simulink model "distributed_swarm_controller"  (R2018a)
settings: Solver=VariableStepAuto  StartTime=0.0  StopTime=Inf  FixedStep=0.01  RelTol=1e-3  EnableMultiTasking=on
model workspace (MAT data in the model file):
  SL_ROS_VariableLengthArrays_MaxSizes.CommonInfo.ArrayTruncateAction = 'EmitWarning'
  SL_ROS_VariableLengthArrays_MaxSizes.MsgTypeMap = containers.Map
  SL_ROS_VariableLengthArrays_MaxSizes.MsgTypeMap.serialization.keys = {'sensor_msgs/Image', 'sensor_msgs/LaserScan'}
  SL_ROS_VariableLengthArrays_MaxSizes.MsgTypeMap.serialization.values{1}(1).PropertyName = 'Data'
  SL_ROS_VariableLengthArrays_MaxSizes.MsgTypeMap.serialization.values{1}(1).DataType = 'uint8'
  SL_ROS_VariableLengthArrays_MaxSizes.MsgTypeMap.serialization.values{1}(1).MaxLength = 691200
  SL_ROS_VariableLengthArrays_MaxSizes.MsgTypeMap.serialization.values{1}(2).PropertyName = 'Encoding'
  SL_ROS_VariableLengthArrays_MaxSizes.MsgTypeMap.serialization.values{1}(2).DataType = 'uint8'
  SL_ROS_VariableLengthArrays_MaxSizes.MsgTypeMap.serialization.values{1}(2).MaxLength = 128
  SL_ROS_VariableLengthArrays_MaxSizes.MsgTypeMap.serialization.values{2}(1).PropertyName = 'Intensities'
  SL_ROS_VariableLengthArrays_MaxSizes.MsgTypeMap.serialization.values{2}(1).DataType = 'single'
  SL_ROS_VariableLengthArrays_MaxSizes.MsgTypeMap.serialization.values{2}(1).MaxLength = 1081
  SL_ROS_VariableLengthArrays_MaxSizes.MsgTypeMap.serialization.values{2}(2).PropertyName = 'Ranges'
  SL_ROS_VariableLengthArrays_MaxSizes.MsgTypeMap.serialization.values{2}(2).DataType = 'single'
  SL_ROS_VariableLengthArrays_MaxSizes.MsgTypeMap.serialization.values{2}(2).MaxLength = 1081
  SL_ROS_VariableLengthArrays_MaxSizes.MsgTypeMap.serialization.uniformity = 0
  SL_ROS_VariableLengthArrays_MaxSizes.MsgTypeMap.serialization.keyType = 'char'
  SL_ROS_VariableLengthArrays_MaxSizes.MsgTypeMap.serialization.valueType = 'any'
undefined symbols (not defined in the file or in its folder): DiscIntNeverNeededParam, Vector_
libraries: robotlib x4, simulink x4, sharedTrackingLibrary x4, aerolibanimutils x1
settings Model: Creator=The MathWorks, Inc.  LastModifiedBy=Kevin_ME813
settings DataIOCC: LimitDataPoints=on  SaveFormat=Array
settings OptimizationCC: LifeSpan=Inf  MaxStackSize=64
settings DebuggingCC: SolverPrmCheckMsg=warning  SFUnexpectedBacktrackingDiag=warning  SFNoUnconditionalDefaultTransitionDiag=warning  SFExecutionAtInitializationDiag=none
settings HardwareCC: ProdBitPerPointer=32  ProdBitPerSizeT=32  ProdBitPerPtrDiffT=32  ProdLargestAtomicFloat=None  ProdIntDivRoundTo=Undefined  ProdEndianess=Unspecified  ProdWordSize=32  ProdHWDeviceType=Generic->Unspecified (assume 32-bit Generic)  UseEmbeddedCoderFeatures=off
settings ModelReferenceCC: PropagateSignalLabelsOutOfModel=off
settings RTWCC: SystemTargetFile=ert.tlc  HardwareBoard=Robot Operating System (ROS)  TLCOptions=-aInlineSetEventsForThisBaseRateFcn=TLC_FALSE -aSuppressMultiTaskScheduler=TLC_FALSE -aRateBasedStepFcn=0  TemplateMakefile=ert_default_tmf  Toolchain=Catkin  TargetLang=C++
settings CodeAppCC: StateflowObjectComments=on
settings ERTTargetCC: MultiwordLength=2048  ERTCustomFileBanners=off  SupportContinuousTime=on  SupportNonInlinedSFcns=on  RemoveResetFunc=off  SupportVariableSizeSignals=on  ModelStepFunctionPrototypeControlCompliant=off  ConvertIfToSwitch=off  SuppressUnreachableDefaultCases=off
settings ConfigComp: CovMetricSettings=dw  CovHtmlReporting=on  CovSaveCumulativeToWorkspaceVar=on  CovSaveSingleToWorkspaceVar=on  CovExternalEMLEnable=off  CovSFcnEnable=off

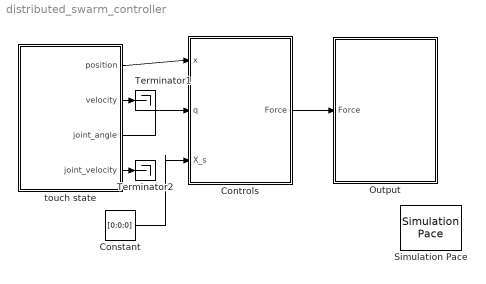
== system distributed_swarm_controller ==
  Constant : Constant  Value=[0;0;0]  SampleTime=0.01
  Controls : Subsystem
  Output : Subsystem
  Simulation Pace : aerolibanimutils/Simulation Pace  SimulationPace=1  SleepMode=MATLAB Thread  OutputPaceError=off  SampleTime=-1
  Terminator1 : Terminator
  Terminator2 : Terminator
  touch state : Subsystem
  wires:
  Controls/1(Force) -> Output/1(Force)
  touch state/1(position) -> Controls/1(x)
  touch state/3(joint_angle) -> Controls/2(q)
  Constant/1 -> Controls/3(X_s)
  touch state/2(velocity) -> Terminator1/1
  touch state/4(joint_velocity) -> Terminator2/1

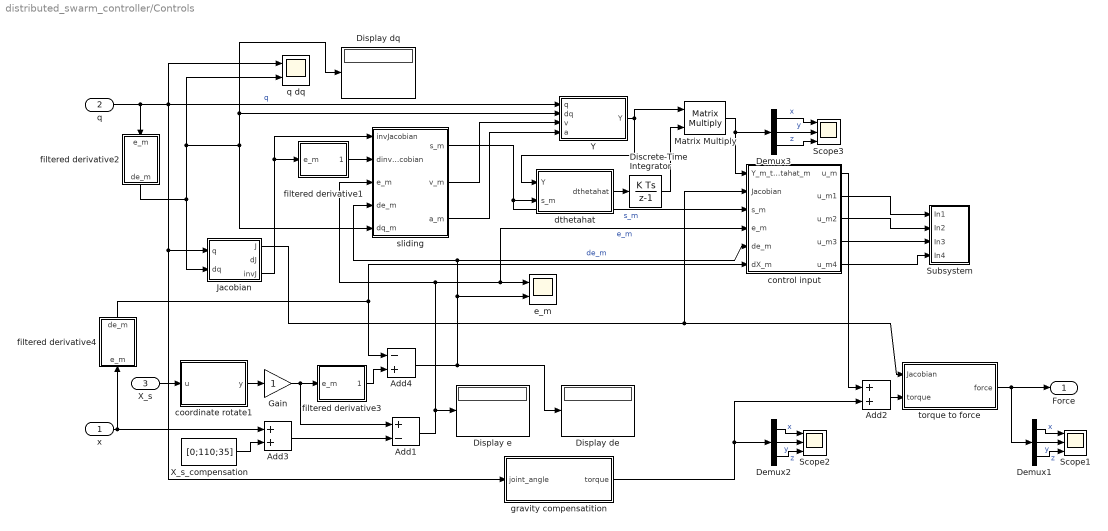
== system distributed_swarm_controller/Controls ==
  x : Inport
  q : Inport  Port=2
  X_s : Inport  Port=3
  Add1 : Sum  Inputs=+-
  Add2 : Sum
  Add3 : Sum
  Add4 : Sum  Inputs=-+
  Demux1 : Demux  Outputs=3
  Demux2 : Demux  Outputs=3
  Demux3 : Demux  Outputs=3
  Discrete-Time Integrator : DiscreteIntegrator  SampleTime=-1  ICPrevOutput=DiscIntNeverNeededParam  ICPrevScaledInput=DiscIntNeverNeededParam
  Display de : Display
  Display dq : Display
  Display e : Display
  Gain : Gain
  Jacobian : MATLAB Function  TreatAsAtomicUnit=on
  Matrix Multiply : Product  Multiplication=Matrix(*)
  Scope1 : Scope  NumInputPorts=3
  Scope2 : Scope  NumInputPorts=3
  Scope3 : Scope  NumInputPorts=3
  Subsystem : Subsystem
  X_s_compensation : Constant  Value=[0;110;35]  SampleTime=0.01
  Y : MATLAB Function  TreatAsAtomicUnit=on
  control input : MATLAB Function  TreatAsAtomicUnit=on
  coordinate rotate1 : MATLAB Function  TreatAsAtomicUnit=on
  dthetahat : MATLAB Function  TreatAsAtomicUnit=on
  e_m : Scope  NumInputPorts=2
  filtered derivative1 : Subsystem
  filtered derivative2 : Subsystem
  filtered derivative3 : Subsystem
  filtered derivative4 : Subsystem
  gravity compensatition : MATLAB Function  TreatAsAtomicUnit=on
  q dq : Scope  NumInputPorts=2
  sliding : MATLAB Function  TreatAsAtomicUnit=on
  torque to force : MATLAB Function  TreatAsAtomicUnit=on
  Force : Outport
  wires:
  Jacobian/1(J) -> torque to force/1(Jacobian), control input/2(Jacobian)
  gravity compensatition/1(torque) -> Demux2/1, Add2/2
  torque to force/1(force) -> Demux1/1, Force/1
  Demux1/1 -> Scope1/1  "x"
  Demux1/3 -> Scope1/3  "z"
  Demux1/2 -> Scope1/2  "y"
  Demux2/2 -> Scope2/2  "y"
  Demux2/3 -> Scope2/3  "z"
  Demux2/1 -> Scope2/1  "x"
  sliding/1(s_m) -> dthetahat/2(s_m), control input/3(s_m)  "s_m"
  q/1 -> Y/1(q), q dq/1, gravity compensatition/1(joint_angle), Jacobian/1(q), filtered derivative2/1(e_m)  "q"
  dthetahat/1(dthetahat) -> Discrete-Time Integrator/1
  Y/1(Y) -> Matrix Multiply/1, dthetahat/1(Y)
  Discrete-Time Integrator/1 -> Matrix Multiply/2
  filtered derivative2/1(de_m) -> Jacobian/2(dq), Display dq/1, Y/2(dq), sliding/5(dq_m), q dq/2
  X_s/1 -> coordinate rotate1/1(u)
  Gain/1 -> filtered derivative3/1(e_m), Add1/1
  coordinate rotate1/1(y) -> Gain/1
  x/1 -> Add3/1, filtered derivative4/1(e_m)
  Add1/1 -> Display e/1, control input/4(e_m), e_m/1, sliding/3(e_m)  "e_m"
  Add4/1 -> Display de/1, e_m/2, control input/5(de_m), sliding/4(de_m)  "de_m"
  control input/1(u_m) -> Add2/1
  Add2/1 -> torque to force/2(torque)
  X_s_compensation/1 -> Add3/2
  Add3/1 -> Add1/2
  filtered derivative3/1(de_m) -> Add4/2
  filtered derivative4/1(de_m) -> control input/6(dX_m), Add4/1
  sliding/2(v_m) -> Y/3(v)
  sliding/3(a_m) -> Y/4(a)
  Jacobian/3(invJ) -> filtered derivative1/1(e_m), sliding/1(invJacobian)
  filtered derivative1/1(de_m) -> sliding/2(dinvJacobian)
  Demux3/2 -> Scope3/2  "y"
  Demux3/3 -> Scope3/3  "z"
  Demux3/1 -> Scope3/1  "x"
  Matrix Multiply/1 -> control input/1(Y_m_thetahat_m), Demux3/1
  control input/2(u_m1) -> Subsystem/1(In1)
  control input/3(u_m2) -> Subsystem/2(In2)
  control input/4(u_m3) -> Subsystem/3(In3)
  control input/5(u_m4) -> Subsystem/4(In4)

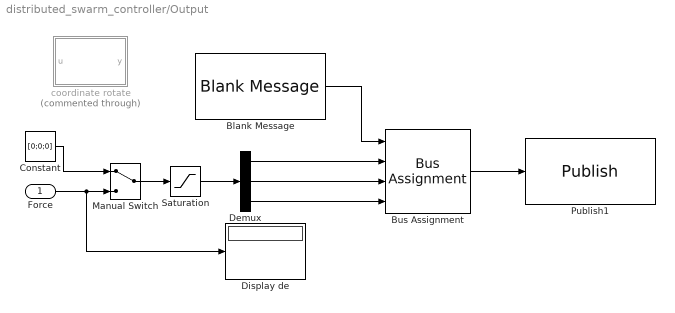
== system distributed_swarm_controller/Output ==
  Force : Inport
  Blank Message : robotlib/Blank Message  SourceLibraryInfo=This block requires Robotics System Toolbox  messageType=geometry_msgs/Vector3Stamped  SampleTime=0.01
      settings: SourceProductBaseCode=RO
  Bus Assignment : BusAssignment  DialogController=Simulink.DDGSource_BusAssignment  AssignedSignals=Vector_.X,Vector_.Y,Vector_.Z
  Constant : Constant  Value=[0;0;0]  SampleTime=0.01
  Demux : Demux  Outputs=3
  Display de : Display
  Manual Switch : ManualSwitch
  Publish1 : robotlib/Publish  SourceLibraryInfo=This block requires Robotics System Toolbox  topicSource=Select from ROS network  topic=/touch_1/touch_force  messageType=geometry_msgs/Vector3Stamped  messageQueueLength=105
      settings: SourceProductBaseCode=RO
  Saturation : Saturate  UpperLimit=[1;1;1]*5  LowerLimit=[-1;-1;-1]*5
  coordinate rotate : MATLAB Function  Commented=through  TreatAsAtomicUnit=on
  wires:
  Demux/2 -> Bus Assignment/3
  Demux/1 -> Bus Assignment/2
  Demux/3 -> Bus Assignment/4
  Bus Assignment/1 -> Publish1/1
  Blank Message/1 -> Bus Assignment/1
  Force/1 -> Display de/1, Manual Switch/2
  Constant/1 -> Manual Switch/1
  Manual Switch/1 -> Saturation/1
  Saturation/1 -> Demux/1

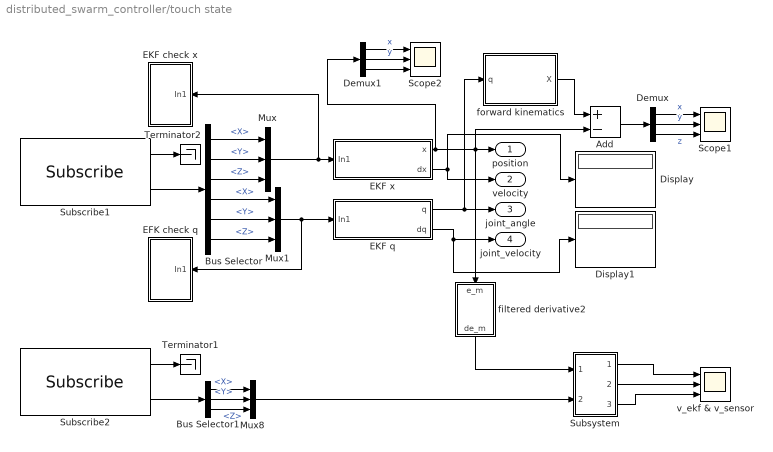
== system distributed_swarm_controller/touch state ==
  Add : Sum  Inputs=+-
  Bus Selector : BusSelector  DialogController=Simulink.DDGSource_BusSelector  OutputSignals=Twist.Linear.X,Twist.Linear.Y,Twist.Linear.Z,Twist.Angular.X,Twist.Angular.Y,Twist.Angular.Z
  Bus Selector1 : BusSelector  DialogController=Simulink.DDGSource_BusSelector  OutputSignals=Vector_.X,Vector_.Y,Vector_.Z
  Demux : Demux  Outputs=3
  Demux1 : Demux  Outputs=3
  Display : Display
  Display1 : Display
  EFK check q : Subsystem
  EKF check x : Subsystem
  EKF q : Subsystem
  EKF x : Subsystem
  Mux : Mux  Inputs=3
  Mux1 : Mux  Inputs=3
  Mux8 : Mux  Inputs=3
  Scope1 : Scope  NumInputPorts=3
  Scope2 : Scope  NumInputPorts=3
  Subscribe1 : robotlib/Subscribe  SourceLibraryInfo=This block requires Robotics System Toolbox  topicSource=Select from ROS network  topic=/touch_1/touch_state  messageType=geometry_msgs/TwistStamped  sampleTime=0.01  messageQueueLength=51
      settings: SourceProductBaseCode=RO
  Subscribe2 : robotlib/Subscribe  SourceLibraryInfo=This block requires Robotics System Toolbox  topicSource=Select from ROS network  topic=/touch_1/touch_vel_hd  messageType=geometry_msgs/Vector3Stamped  sampleTime=0.01  messageQueueLength=51
      settings: SourceProductBaseCode=RO
  Subsystem : Subsystem
  Terminator1 : Terminator
  Terminator2 : Terminator
  filtered derivative2 : Subsystem
  forward kinematics : MATLAB Function  TreatAsAtomicUnit=on
  v_ekf & v_sensor : Scope  NumInputPorts=3
  position : Outport
  velocity : Outport  Port=2
  joint_angle : Outport  Port=3
  joint_velocity : Outport  Port=4
  wires:
  Subscribe1/2 -> Bus Selector/1
  Bus Selector/1 -> Mux/1  "<X>"
  Bus Selector/5 -> Mux1/2  "<Y>"
  Bus Selector/4 -> Mux1/1  "<X>"
  Bus Selector/6 -> Mux1/3  "<Z>"
  Add/1 -> Demux/1
  Demux/3 -> Scope1/3  "z"
  Demux/1 -> Scope1/1  "x"
  Demux/2 -> Scope1/2  "y"
  Subscribe2/1 -> Terminator1/1
  Subscribe1/1 -> Terminator2/1
  Mux1/1 -> EFK check q/1(In1), EKF q/1(In1)
  Subscribe2/2 -> Bus Selector1/1
  forward kinematics/1(X) -> Add/1
  Bus Selector/2 -> Mux/2  "<Y>"
  Bus Selector/3 -> Mux/3  "<Z>"
  Mux/1 -> EKF x/1(In1), EKF check x/1(In1)
  EKF q/1(q) -> forward kinematics/1(q), joint_angle/1
  EKF x/2(dx) -> velocity/1, Display/1
  EKF q/2(dq) -> Display1/1, joint_velocity/1
  Subsystem/1(Out1) -> v_ekf & v_sensor/1
  Subsystem/2(Out2) -> v_ekf & v_sensor/2
  Subsystem/3(Out3) -> v_ekf & v_sensor/3
  Bus Selector1/1 -> Mux8/1  "<X>"
  Bus Selector1/2 -> Mux8/2  "<Y>"
  Bus Selector1/3 -> Mux8/3  "<Z>"
  Mux8/1 -> Subsystem/2(In2)
  filtered derivative2/1(de_m) -> Subsystem/1(In1)
  Demux1/2 -> Scope2/2  "y"
  Demux1/1 -> Scope2/1  "x"
  EKF x/1(x) -> Demux1/1, filtered derivative2/1(e_m), position/1, Add/2
  Demux1/3 -> Scope2/3

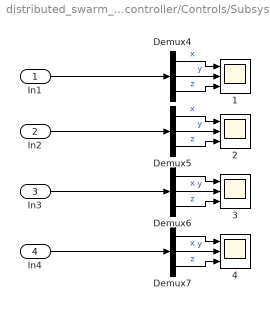
== system distributed_swarm_controller/Controls/Subsystem ==
  In1 : Inport
  In2 : Inport  Port=2
  In3 : Inport  Port=3
  In4 : Inport  Port=4
  {1..4} (4 alike) : Scope  NumInputPorts=3
  Demux{4..7} (4 alike) : Demux  Outputs=3
  wires:
  Demux5/1 -> 2/1  "x"
  Demux6/3 -> 3/3  "z"
  Demux6/1 -> 3/1  "x"
  In4/1 -> Demux7/1
  Demux5/3 -> 2/3  "z"
  Demux4/3 -> 1/3  "z"
  Demux6/2 -> 3/2  "y"
  Demux5/2 -> 2/2  "y"
  Demux4/2 -> 1/2  "y"
  Demux4/1 -> 1/1  "x"
  Demux7/1 -> 4/1  "x"
  Demux7/3 -> 4/3  "z"
  In2/1 -> Demux5/1
  Demux7/2 -> 4/2  "y"
  In3/1 -> Demux6/1
  In1/1 -> Demux4/1

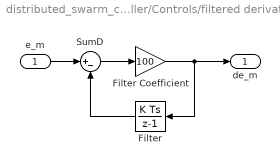
== system distributed_swarm_controller/Controls/filtered derivative1 ==
  e_m : Inport
  Filter : DiscreteIntegrator  DisableCoverage=on  SampleTime=-1  ICPrevOutput=DiscIntNeverNeededParam  ICPrevScaledInput=DiscIntNeverNeededParam
  Filter Coefficient : Gain  Gain=100
  SumD : Sum  DisableCoverage=on  Inputs=|+-
  de_m : Outport
  wires:
  e_m/1 -> SumD/1
  SumD/1 -> Filter Coefficient/1
  Filter/1 -> SumD/2
  Filter Coefficient/1 -> Filter/1, de_m/1

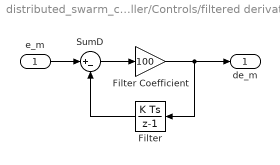
== system distributed_swarm_controller/Controls/filtered derivative2 ==
  e_m : Inport
  Filter : DiscreteIntegrator  DisableCoverage=on  SampleTime=-1  ICPrevOutput=DiscIntNeverNeededParam  ICPrevScaledInput=DiscIntNeverNeededParam
  Filter Coefficient : Gain  Gain=100
  SumD : Sum  DisableCoverage=on  Inputs=|+-
  de_m : Outport
  wires:
  Filter Coefficient/1 -> de_m/1, Filter/1
  Filter/1 -> SumD/2
  SumD/1 -> Filter Coefficient/1
  e_m/1 -> SumD/1

== system distributed_swarm_controller/Controls/filtered derivative3 ==
  e_m : Inport
  Filter : DiscreteIntegrator  DisableCoverage=on  SampleTime=-1  ICPrevOutput=DiscIntNeverNeededParam  ICPrevScaledInput=DiscIntNeverNeededParam
  Filter Coefficient : Gain  Gain=100
  SumD : Sum  DisableCoverage=on  Inputs=|+-
  de_m : Outport
  wires:
  Filter Coefficient/1 -> de_m/1, Filter/1
  Filter/1 -> SumD/2
  SumD/1 -> Filter Coefficient/1
  e_m/1 -> SumD/1

== system distributed_swarm_controller/Controls/filtered derivative4 ==
  e_m : Inport
  Filter : DiscreteIntegrator  DisableCoverage=on  SampleTime=-1  ICPrevOutput=DiscIntNeverNeededParam  ICPrevScaledInput=DiscIntNeverNeededParam
  Filter Coefficient : Gain  Gain=100
  SumD : Sum  DisableCoverage=on  Inputs=|+-
  de_m : Outport
  wires:
  e_m/1 -> SumD/1
  SumD/1 -> Filter Coefficient/1
  Filter/1 -> SumD/2
  Filter Coefficient/1 -> Filter/1, de_m/1

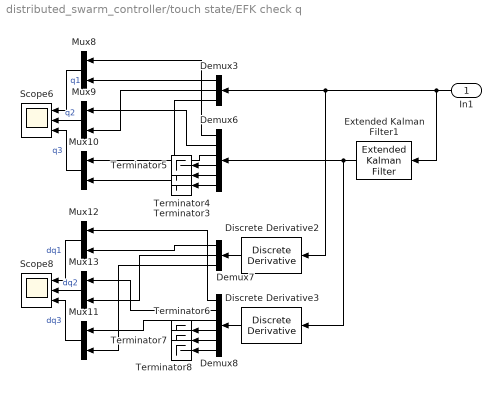
== system distributed_swarm_controller/touch state/EFK check q ==
  In1 : Inport
  Demux3 : Demux  Outputs=3
  Demux6 : Demux  Outputs=6
  Demux7 : Demux  Outputs=3
  Demux8 : Demux  Outputs=6
  Discrete Derivative2 : simulink/Discrete/Discrete Derivative  gainval=1.0  ICPrevScaledInput=0.0  OutMin=[]  OutMax=[]  OutDataType=fixdt(1, 16)  OutScaling=2^-10  DoSatur=off
  Discrete Derivative3 : simulink/Discrete/Discrete Derivative  gainval=1.0  ICPrevScaledInput=0.0  OutMin=[]  OutMax=[]  OutDataType=fixdt(1, 16)  OutScaling=2^-10  DoSatur=off
  Extended Kalman Filter1 : sharedTrackingLibrary/Extended Kalman Filter  StateTransitionFcn=myStateTransitionFcn  HasStateTransitionJacobianFcn=off  HasAdditiveProcessNoise=Additive  ProcessNoise=diag([0 0 0 1 1 1]*1e-3)  HasTimeVaryingProcessNoise=off  HasStateTransitionFcnExtraArgument=0  InitialState=[0 0 0 0 0 0]  InitialStateCovariance=1e-2  MeasurementFcn1=myMeasurementFcn  HasMeasurementJacobianFcn1=off  HasMeasurementEnablePort1=off  HasAdditiveMeasurementNoise1=Additive  MeasurementNoise1=diag([1;1;1]*1e-2)  HasTimeVaryingMeasurementNoise1=off  HasMeasurementFcnExtraArgument1=0  MeasurementFcn2=myMeasurementFcn  HasMeasurementJacobianFcn2=off  HasMeasurementEnablePort2=off  HasAdditiveMeasurementNoise2=Additive  MeasurementNoise2=1  HasTimeVaryingMeasurementNoise2=off  HasMeasurementFcnExtraArgument2=0  MeasurementFcn3=myMeasurementFcn  HasMeasurementJacobianFcn3=off  HasMeasurementEnablePort3=off  HasAdditiveMeasurementNoise3=Additive  MeasurementNoise3=1  HasTimeVaryingMeasurementNoise3=off  HasMeasurementFcnExtraArgument3=0  MeasurementFcn4=myMeasurementFcn  HasMeasurementJacobianFcn4=off  HasMeasurementEnablePort4=off  HasAdditiveMeasurementNoise4=Additive  MeasurementNoise4=1  HasTimeVaryingMeasurementNoise4=off  HasMeasurementFcnExtraArgument4=0  MeasurementFcn5=myMeasurementFcn  HasMeasurementJacobianFcn5=off  HasMeasurementEnablePort5=off  HasAdditiveMeasurementNoise5=Additive  MeasurementNoise5=1  HasTimeVaryingMeasurementNoise5=off  HasMeasurementFcnExtraArgument5=0  EnableMultirate=off  StateTransitionFcnSampleTime=1  MeasurementFcn1SampleTime=1  MeasurementFcn2SampleTime=1  MeasurementFcn3SampleTime=1  MeasurementFcn4SampleTime=1  MeasurementFcn5SampleTime=1  UseCurrentEstimator=on  OutputStateCovariance=off  DataType=double  SampleTime=0.01  NumberOfMeasurements=1
      settings: SourceProductName=Control System Toolbox  SourceProductBaseCode=CT
  Mux{8..13} (6 alike) : Mux  Inputs=2
  Scope6 : Scope  NumInputPorts=3
  Scope8 : Scope  NumInputPorts=3
  Terminator{3..8} (6 alike) : Terminator
  wires:
  In1/1 -> Discrete Derivative2/1, Demux3/1, Extended Kalman Filter1/1
  Demux3/1 -> Mux8/2
  Demux8/3 -> Mux11/1
  Demux3/2 -> Mux9/2
  Mux11/1 -> Scope8/3  "dq3"
  Mux12/1 -> Scope8/1  "dq1"
  Demux3/3 -> Mux10/2
  Demux7/2 -> Mux13/2
  Demux6/4 -> Terminator5/1
  Demux6/2 -> Mux9/1
  Demux8/5 -> Terminator7/1
  Demux8/4 -> Terminator6/1
  Mux13/1 -> Scope8/2  "dq2"
  Demux8/1 -> Mux12/1
  Mux9/1 -> Scope6/2  "q2"
  Mux10/1 -> Scope6/3  "q3"
  Demux6/3 -> Mux10/1
  Mux8/1 -> Scope6/1  "q1"
  Demux8/2 -> Mux13/1
  Demux6/1 -> Mux8/1
  Demux8/6 -> Terminator8/1
  Extended Kalman Filter1/1 -> Demux6/1, Discrete Derivative3/1
  Demux6/5 -> Terminator4/1
  Demux7/1 -> Mux12/2
  Demux7/3 -> Mux11/2
  Discrete Derivative2/1 -> Demux7/1
  Demux6/6 -> Terminator3/1
  Discrete Derivative3/1 -> Demux8/1

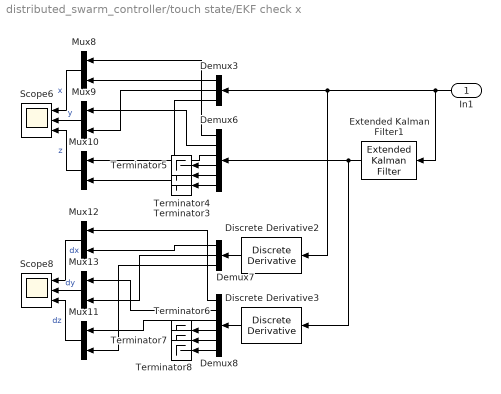
== system distributed_swarm_controller/touch state/EKF check x ==
  In1 : Inport
  Demux3 : Demux  Outputs=3
  Demux6 : Demux  Outputs=6
  Demux7 : Demux  Outputs=3
  Demux8 : Demux  Outputs=6
  Discrete Derivative2 : simulink/Discrete/Discrete Derivative  gainval=1.0  ICPrevScaledInput=0.0  OutMin=[]  OutMax=[]  OutDataType=fixdt(1, 16)  OutScaling=2^-10  DoSatur=off
  Discrete Derivative3 : simulink/Discrete/Discrete Derivative  gainval=1.0  ICPrevScaledInput=0.0  OutMin=[]  OutMax=[]  OutDataType=fixdt(1, 16)  OutScaling=2^-10  DoSatur=off
  Extended Kalman Filter1 : sharedTrackingLibrary/Extended Kalman Filter  StateTransitionFcn=myStateTransitionFcn  HasStateTransitionJacobianFcn=off  HasAdditiveProcessNoise=Additive  ProcessNoise=diag([0 0 0 1 1 1]*1e-3)  HasTimeVaryingProcessNoise=off  HasStateTransitionFcnExtraArgument=0  InitialState=[0 0 0 0 0 0]  InitialStateCovariance=1e-2  MeasurementFcn1=myMeasurementFcn  HasMeasurementJacobianFcn1=off  HasMeasurementEnablePort1=off  HasAdditiveMeasurementNoise1=Additive  MeasurementNoise1=diag([1;1;1]*1e-2)  HasTimeVaryingMeasurementNoise1=off  HasMeasurementFcnExtraArgument1=0  MeasurementFcn2=myMeasurementFcn  HasMeasurementJacobianFcn2=off  HasMeasurementEnablePort2=off  HasAdditiveMeasurementNoise2=Additive  MeasurementNoise2=1  HasTimeVaryingMeasurementNoise2=off  HasMeasurementFcnExtraArgument2=0  MeasurementFcn3=myMeasurementFcn  HasMeasurementJacobianFcn3=off  HasMeasurementEnablePort3=off  HasAdditiveMeasurementNoise3=Additive  MeasurementNoise3=1  HasTimeVaryingMeasurementNoise3=off  HasMeasurementFcnExtraArgument3=0  MeasurementFcn4=myMeasurementFcn  HasMeasurementJacobianFcn4=off  HasMeasurementEnablePort4=off  HasAdditiveMeasurementNoise4=Additive  MeasurementNoise4=1  HasTimeVaryingMeasurementNoise4=off  HasMeasurementFcnExtraArgument4=0  MeasurementFcn5=myMeasurementFcn  HasMeasurementJacobianFcn5=off  HasMeasurementEnablePort5=off  HasAdditiveMeasurementNoise5=Additive  MeasurementNoise5=1  HasTimeVaryingMeasurementNoise5=off  HasMeasurementFcnExtraArgument5=0  EnableMultirate=off  StateTransitionFcnSampleTime=1  MeasurementFcn1SampleTime=1  MeasurementFcn2SampleTime=1  MeasurementFcn3SampleTime=1  MeasurementFcn4SampleTime=1  MeasurementFcn5SampleTime=1  UseCurrentEstimator=on  OutputStateCovariance=off  DataType=double  SampleTime=0.01  NumberOfMeasurements=1
      settings: SourceProductName=Control System Toolbox  SourceProductBaseCode=CT
  Mux{8..13} (6 alike) : Mux  Inputs=2
  Scope6 : Scope  NumInputPorts=3
  Scope8 : Scope  NumInputPorts=3
  Terminator{3..8} (6 alike) : Terminator
  wires:
  Discrete Derivative3/1 -> Demux8/1
  Demux6/6 -> Terminator3/1
  Discrete Derivative2/1 -> Demux7/1
  Demux7/3 -> Mux11/2
  Demux7/1 -> Mux12/2
  Demux6/5 -> Terminator4/1
  Extended Kalman Filter1/1 -> Demux6/1, Discrete Derivative3/1
  Demux8/6 -> Terminator8/1
  Demux6/1 -> Mux8/1
  Demux8/2 -> Mux13/1
  Mux8/1 -> Scope6/1  "x"
  Demux6/3 -> Mux10/1
  Mux10/1 -> Scope6/3  "z"
  Mux9/1 -> Scope6/2  "y"
  Demux8/1 -> Mux12/1
  Mux13/1 -> Scope8/2  "dy"
  Demux8/4 -> Terminator6/1
  Demux8/5 -> Terminator7/1
  Demux6/2 -> Mux9/1
  Demux6/4 -> Terminator5/1
  Demux7/2 -> Mux13/2
  Demux3/3 -> Mux10/2
  Mux12/1 -> Scope8/1  "dx"
  Mux11/1 -> Scope8/3  "dz"
  Demux3/2 -> Mux9/2
  Demux8/3 -> Mux11/1
  Demux3/1 -> Mux8/2
  In1/1 -> Extended Kalman Filter1/1, Demux3/1, Discrete Derivative2/1

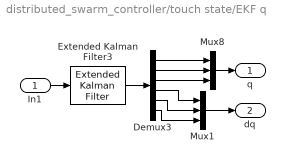
== system distributed_swarm_controller/touch state/EKF q ==
  In1 : Inport
  Demux3 : Demux  Outputs=6
  Extended Kalman Filter3 : sharedTrackingLibrary/Extended Kalman Filter  StateTransitionFcn=myStateTransitionFcn  HasStateTransitionJacobianFcn=off  HasAdditiveProcessNoise=Additive  ProcessNoise=diag([0 0 0 1 1 1]*5e-2)  HasTimeVaryingProcessNoise=off  HasStateTransitionFcnExtraArgument=0  InitialState=[0 0 0 0 0 0]  InitialStateCovariance=diag([1 1 1 1 1 1]*1e-1)  MeasurementFcn1=myMeasurementFcn  HasMeasurementJacobianFcn1=off  HasMeasurementEnablePort1=off  HasAdditiveMeasurementNoise1=Additive  MeasurementNoise1=diag([1;1;1]*3e-3)  HasTimeVaryingMeasurementNoise1=off  HasMeasurementFcnExtraArgument1=0  MeasurementFcn2=myMeasurementFcn  HasMeasurementJacobianFcn2=off  HasMeasurementEnablePort2=off  HasAdditiveMeasurementNoise2=Additive  MeasurementNoise2=1  HasTimeVaryingMeasurementNoise2=off  HasMeasurementFcnExtraArgument2=0  MeasurementFcn3=myMeasurementFcn  HasMeasurementJacobianFcn3=off  HasMeasurementEnablePort3=off  HasAdditiveMeasurementNoise3=Additive  MeasurementNoise3=1  HasTimeVaryingMeasurementNoise3=off  HasMeasurementFcnExtraArgument3=0  MeasurementFcn4=myMeasurementFcn  HasMeasurementJacobianFcn4=off  HasMeasurementEnablePort4=off  HasAdditiveMeasurementNoise4=Additive  MeasurementNoise4=1  HasTimeVaryingMeasurementNoise4=off  HasMeasurementFcnExtraArgument4=0  MeasurementFcn5=myMeasurementFcn  HasMeasurementJacobianFcn5=off  HasMeasurementEnablePort5=off  HasAdditiveMeasurementNoise5=Additive  MeasurementNoise5=1  HasTimeVaryingMeasurementNoise5=off  HasMeasurementFcnExtraArgument5=0  EnableMultirate=off  StateTransitionFcnSampleTime=1  MeasurementFcn1SampleTime=1  MeasurementFcn2SampleTime=1  MeasurementFcn3SampleTime=1  MeasurementFcn4SampleTime=1  MeasurementFcn5SampleTime=1  UseCurrentEstimator=on  OutputStateCovariance=off  DataType=double  SampleTime=0.01  NumberOfMeasurements=1
      settings: SourceProductName=Control System Toolbox  SourceProductBaseCode=CT
  Mux1 : Mux  Inputs=3
  Mux8 : Mux  Inputs=3
  q : Outport
  dq : Outport  Port=2
  wires:
  Mux8/1 -> q/1
  Demux3/6 -> Mux1/3
  Demux3/2 -> Mux8/2
  Demux3/3 -> Mux8/3
  Demux3/1 -> Mux8/1
  In1/1 -> Extended Kalman Filter3/1
  Demux3/4 -> Mux1/1
  Extended Kalman Filter3/1 -> Demux3/1
  Demux3/5 -> Mux1/2
  Mux1/1 -> dq/1

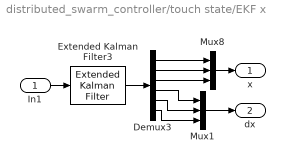
== system distributed_swarm_controller/touch state/EKF x ==
  In1 : Inport
  Demux3 : Demux  Outputs=6
  Extended Kalman Filter3 : sharedTrackingLibrary/Extended Kalman Filter  StateTransitionFcn=myStateTransitionFcn  HasStateTransitionJacobianFcn=off  HasAdditiveProcessNoise=Additive  ProcessNoise=diag([0 0 0 1 1 1]*5e-2)  HasTimeVaryingProcessNoise=off  HasStateTransitionFcnExtraArgument=0  InitialState=[4 -110 -35 0 0 0]  InitialStateCovariance=diag([2 1 2 1 1 1])  MeasurementFcn1=myMeasurementFcn  HasMeasurementJacobianFcn1=off  HasMeasurementEnablePort1=off  HasAdditiveMeasurementNoise1=Additive  MeasurementNoise1=diag([1;1;1]*3e-3)  HasTimeVaryingMeasurementNoise1=off  HasMeasurementFcnExtraArgument1=0  MeasurementFcn2=myMeasurementFcn  HasMeasurementJacobianFcn2=off  HasMeasurementEnablePort2=off  HasAdditiveMeasurementNoise2=Additive  MeasurementNoise2=1  HasTimeVaryingMeasurementNoise2=off  HasMeasurementFcnExtraArgument2=0  MeasurementFcn3=myMeasurementFcn  HasMeasurementJacobianFcn3=off  HasMeasurementEnablePort3=off  HasAdditiveMeasurementNoise3=Additive  MeasurementNoise3=1  HasTimeVaryingMeasurementNoise3=off  HasMeasurementFcnExtraArgument3=0  MeasurementFcn4=myMeasurementFcn  HasMeasurementJacobianFcn4=off  HasMeasurementEnablePort4=off  HasAdditiveMeasurementNoise4=Additive  MeasurementNoise4=1  HasTimeVaryingMeasurementNoise4=off  HasMeasurementFcnExtraArgument4=0  MeasurementFcn5=myMeasurementFcn  HasMeasurementJacobianFcn5=off  HasMeasurementEnablePort5=off  HasAdditiveMeasurementNoise5=Additive  MeasurementNoise5=1  HasTimeVaryingMeasurementNoise5=off  HasMeasurementFcnExtraArgument5=0  EnableMultirate=off  StateTransitionFcnSampleTime=1  MeasurementFcn1SampleTime=1  MeasurementFcn2SampleTime=1  MeasurementFcn3SampleTime=1  MeasurementFcn4SampleTime=1  MeasurementFcn5SampleTime=1  UseCurrentEstimator=on  OutputStateCovariance=off  DataType=double  SampleTime=0.01  NumberOfMeasurements=1
      settings: SourceProductName=Control System Toolbox  SourceProductBaseCode=CT
  Mux1 : Mux  Inputs=3
  Mux8 : Mux  Inputs=3
  x : Outport
  dx : Outport  Port=2
  wires:
  Demux3/5 -> Mux1/2
  Extended Kalman Filter3/1 -> Demux3/1
  Demux3/4 -> Mux1/1
  In1/1 -> Extended Kalman Filter3/1
  Demux3/1 -> Mux8/1
  Demux3/3 -> Mux8/3
  Demux3/2 -> Mux8/2
  Demux3/6 -> Mux1/3
  Mux8/1 -> x/1
  Mux1/1 -> dx/1

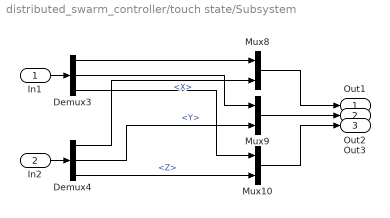
== system distributed_swarm_controller/touch state/Subsystem ==
  In1 : Inport
  In2 : Inport  Port=2
  Demux3 : Demux  Outputs=3
  Demux4 : Demux  Outputs=3
  Mux10 : Mux  Inputs=2
  Mux8 : Mux  Inputs=2
  Mux9 : Mux  Inputs=2
  Out1 : Outport
  Out2 : Outport  Port=2
  Out3 : Outport  Port=3
  wires:
  In2/1 -> Demux4/1
  Demux4/2 -> Mux9/2  "<Y>"
  Demux3/1 -> Mux8/1
  Demux4/1 -> Mux8/2  "<X>"
  Demux3/3 -> Mux10/1
  Demux3/2 -> Mux9/1
  Mux10/1 -> Out3/1
  Demux4/3 -> Mux10/2  "<Z>"
  Mux8/1 -> Out1/1
  Mux9/1 -> Out2/1
  In1/1 -> Demux3/1

== system distributed_swarm_controller/touch state/filtered derivative2 ==
  e_m : Inport
  Filter : DiscreteIntegrator  DisableCoverage=on  SampleTime=-1  ICPrevOutput=DiscIntNeverNeededParam  ICPrevScaledInput=DiscIntNeverNeededParam
  Filter Coefficient : Gain  Gain=100
  SumD : Sum  DisableCoverage=on  Inputs=|+-
  de_m : Outport
  wires:
  Filter Coefficient/1 -> de_m/1, Filter/1
  Filter/1 -> SumD/2
  SumD/1 -> Filter Coefficient/1
  e_m/1 -> SumD/1

== matlab function distributed_swarm_controller/Controls/torque to force ==
  data: Jacobian input; torque input; force output
function force = fcn(Jacobian, torque)

force = pinv(Jacobian).'*torque;

== matlab function distributed_swarm_controller/Controls/gravity compensatition ==
  data: joint_angle input; torque output
function torque = fcn(joint_angle)
q1 = joint_angle(1);
q2 = joint_angle(2);
q3 = joint_angle(3);
c1 = 85;
c2 = 70;

result = [0;c1*sin(q2+q3)+c2*cos(q2);c1*sin(q2+q3)];
% if result(2) < 0
%     result(2) = 0;
% end
torque = result;

== matlab function distributed_swarm_controller/touch state/forward kinematics ==
  data: q input; X output
function X = fcn(q)
%#codegen

l1=133;
l2=133;

q1 = q(1);
q2 = q(2);
q3 = q(3);

s1 = sin(q1);
s2 = sin(q2);
s3 = sin(q3);

c1 = cos(q1);
c2 = cos(q2);
c3 = cos(q3);

X1 = -l1*s1*c2 - l2*s1*s2*c3 - l2*s1*c2*s3;
X2 = l1*s2 - l2*c2*c3 + l2*s2*s3 + l2;
X3 = l1*c1*c2 - l1 + l2*c1*s2*c3 + l2*c1*c2*s3;

X = [ X1;
      X2;
      X3];

== matlab function distributed_swarm_controller/Output/coordinate rotate ==
  data: u input; y output
function y = fcn(u)

y = roty(-90)*rotx(-90)*u;

== matlab function distributed_swarm_controller/Controls/control input ==
  data: Y_m_thetahat_m input; Jacobian input; s_m input; e_m input; u_m output; de_m input; dX_m input; u_m1 output; u_m2 output; u_m3 output; u_m4 output
function [u_m, u_m1,u_m2, u_m3, u_m4] = fcn(Y_m_thetahat_m, Jacobian, s_m, e_m, de_m, dX_m)
k_sm = diag([15;20;20]);
k_pm = diag([1.7;2.5;2.5]*10^(-4));
k_dm = diag([1.7;1.5;1.5]*10^(-4));
k_tm = diag([1;1.5;1.5]*4);
p_m = -k_tm*e_m + dX_m;
% u_m = Y_m_thetahat_m ...
%     - (k_sm + k_pm*Jacobian.'*Jacobian)*s_m ...
%     + k_dm*Jacobian.'*de_m;
u_m1 = Y_m_thetahat_m;
u_m2 = - k_sm*s_m;
u_m3 = - k_pm*Jacobian.'*p_m;
u_m4 = k_dm*Jacobian.'*de_m;
u_m = u_m1 + u_m2 + u_m3 + u_m4;

== matlab function distributed_swarm_controller/Controls/sliding ==
  data: invJacobian input; dinvJacobian input; e_m input; de_m input; dq_m input; s_m output; v_m output; a_m output
function [s_m, v_m, a_m] = fcn(invJacobian, dinvJacobian, e_m, de_m, dq_m)
k_tm = diag([1;1.5;1.5]*4);
s_m = -invJacobian*k_tm*e_m + dq_m;
v_m = dq_m - s_m;
a_m = dinvJacobian*k_tm*e_m + invJacobian*k_tm*de_m;

== matlab function distributed_swarm_controller/Controls/Y ==
  data: q input; Y output; dq input; v input; a input
function Y = fcn(q,dq,v,a)
%#codegen

Y11=a(1)*cos(2*q(2))-sin(2*q(2))*(v(2)*dq(1)-v(1)*dq(2));
Y12=-sin(2*q(2)+2*q(3))*dq(1)*(v(2)+v(3))-v(1)*sin(2*q(2)+2*q(3))*(dq(2)-dq(3))+a(1)*cos(2*q(2)+2*q(3));
Y13=a(1)*(sin(2*q(2)+ q(3))+sin(q(3)))+0.5*cos(q(3))*(v(1)*dq(3)+v(3)*dq(1))+cos(2*q(2)+q(3))*(v(2)*dq(1)+0.5*v(3)*dq(1)+v(1)*dq(2)+0.5*v(1)*dq(3));
Y14=a(1);
Y15=0;
Y16=0;
Y17=0;
Y18=0;

Y21=v(1)*sin(2*q(2))*dq(1);
Y22=v(1)*sin(2*q(2)+2*q(3))*dq(1);
Y23=sin(q(3))*(2*a(2)+a(3))-v(1)*cos(2*q(2)+q(3))*dq(1)+cos(q(3))*(v(3)*dq(2)+v(3)*dq(3)+v(2)*dq(3));
Y24=0;
Y25=a(2);
Y26=a(3);
Y27=sin(q(2)+q(3));
Y28=cos(q(2));


Y31=0;
Y32=v(1)*sin(2*q(2)+2*q(3))*dq(1);
Y33=a(2)*sin(q(3))-(0.5*v(1)*cos(2*q(2)+q(3))+0.5*v(1)*cos(q(3)))*dq(1)-cos(q(3))*v(2)*dq(2);
Y34=0;
Y35=0;
Y36=a(2)+a(3);
Y37=sin(q(2)+q(3));
Y38=0;

Y = [ Y11 Y21 Y31;
      Y12 Y22 Y32;
      Y13 Y23 Y33;
      Y14 Y24 Y34;
      Y15 Y25 Y35;
      Y16 Y26 Y36;
      Y17 Y27 Y37;
      Y18 Y28 Y38 ].';

== matlab function distributed_swarm_controller/Controls/dthetahat ==
  data: Y input; dthetahat output; s_m input
function dthetahat = fcn(Y, s_m)
%#codegen
dthetahat = -Y.'* s_m;

== matlab function distributed_swarm_controller/Controls/coordinate rotate1 ==
  data: u input; y output
function y = fcn(u)

y = roty(-90)*rotx(-90)*u;

== matlab function distributed_swarm_controller/Controls/Jacobian ==
  data: q input; J output; dJ output; dq input; invJ output
function [J, dJ, invJ] = fcn(q, dq)
%#codegen

L1=133;
L2=133;

q1 = q(1);
q2 = q(2);
q3 = q(3);

dq1 = dq(1);
dq2 = dq(2);
dq3 = dq(3);

j11 = -L1*cos( q1 )*cos( q2 ) - L2*cos( q1 )*cos( q2 )*sin( q3 ) - L2*cos( q1 )*sin( q2 )*cos( q3 );
j12 = L2*sin( q1 )*sin( q2 )*sin( q3 ) + L1*sin( q1 )*sin( q2 ) - L2*sin( q1 )*cos( q2 )*cos( q3 );
j13 = -L2*sin( q1 )*cos( q2 )*cos( q3 ) + L2*sin( q1 )*sin( q2 )*sin( q3 );
j22 = L2*sin( q2 )*cos( q3 ) + L2*cos( q2 )*sin( q3 ) + L1*cos( q(2) );
j23 = L2*cos( q2 )*sin( q3 ) + L2*sin( q2 )*cos( q3 );
j31 = -L2*sin( q1 )*sin( q2 )*cos( q3 ) - L1*sin( q1 )*cos( q2 ) - L2*sin( q1 )*cos( q2 )*sin( q3 );
j32 = L2*cos( q1 )*cos( q2 )*cos( q3 ) - L2*cos( q1 )*sin( q2 )*sin( q3 ) - L1*cos( q1 )*sin( q2 );
j33 = L2*cos( q1 )*cos( q2 )*cos( q3 ) - L2*cos( q1 )*sin( q2 )*sin( q3 );

J = [ j11 j12 j13;
       0  j22 j23;
      j31 j32 j33];

dJ11=L1*dq1*cos( q2 )*sin( q1 ) + L1*dq2*cos( q1 )*sin( q2 ) - L2*dq2*cos( q1 )*cos( q2 )*cos( q3 ) - L2*dq3*cos( q1 )*cos( q2 )*cos( q3 ) + L2*dq1*cos( q2 )*sin( q1 )*sin( q3 ) + L2*dq1*cos( q3 )*sin( q1 )*sin( q2 ) + L2*dq2*cos( q1 )*sin( q2 )*sin( q3 ) + L2*dq3*cos( q1 )*sin( q2 )*sin( q3 );
dJ12=L1*dq1*cos( q1 )*sin( q2 ) + L1*dq2*cos( q2 )*sin( q1 ) - L2*dq1*cos( q1 )*cos( q2 )*cos( q3 ) + L2*dq1*cos( q1 )*sin( q2 )*sin( q3 ) + L2*dq2*cos( q2 )*sin( q1 )*sin( q3 ) + L2*dq2*cos( q3 )*sin( q1 )*sin( q2 ) + L2*dq3*cos( q2 )*sin( q1 )*sin( q3 ) + L2*dq3*cos( q3 )*sin( q1 )*sin( q2 );
dJ13=L2*dq1*cos( q1 )*sin( q2 )*sin( q3 ) - L2*dq1*cos( q1 )*cos( q2 )*cos( q3 ) + L2*dq2*cos( q2 )*sin( q1 )*sin( q3 ) + L2*dq2*cos( q3 )*sin( q1 )*sin( q2 ) + L2*dq3*cos( q2 )*sin( q1 )*sin( q3 ) + L2*dq3*cos( q3 )*sin( q1 )*sin( q2 );
dJ22=L2*dq2*cos( q2 )*cos( q3 ) - L1*dq2*sin( q2 ) + L2*dq3*cos( q2 )*cos( q3 ) - L2*dq2*sin( q2 )*sin( q3 ) - L2*dq3*sin( q2 )*sin( q3 );
dJ23=L2*dq2*cos( q2 )*cos( q3 ) + L2*dq3*cos( q2 )*cos( q3 ) - L2*dq2*sin( q2 )*sin( q3 ) - L2*dq3*sin( q2 )*sin( q3 );
dJ31=L1*dq2*sin( q1 )*sin( q2 ) - L1*dq1*cos( q1 )*cos( q2 ) - L2*dq1*cos( q1 )*cos( q2 )*sin( q3 ) - L2*dq1*cos( q1 )*cos( q3 )*sin( q2 ) - L2*dq2*cos( q2 )*cos( q3 )*sin( q1 ) - L2*dq3*cos( q2 )*cos( q3 )*sin( q1 ) + L2*dq2*sin( q1 )*sin( q2 )*sin( q3 ) + L2*dq3*sin( q1 )*sin( q2 )*sin( q3 );
dJ32=L1*dq1*sin( q1 )*sin( q2 ) - L1*dq2*cos( q1 )*cos( q2 ) - L2*dq1*cos( q2 )*cos( q3 )*sin( q1 ) - L2*dq2*cos( q1 )*cos( q2 )*sin( q3 ) - L2*dq2*cos( q1 )*cos( q3 )*sin( q2 ) - L2*dq3*cos( q1 )*cos( q2 )*sin( q3 ) - L2*dq3*cos( q1 )*cos( q3 )*sin( q2 ) + L2*dq1*sin( q1 )*sin( q2 )*sin( q3 );
dJ33=L2*dq1*sin( q1 )*sin( q2 )*sin( q3 ) - L2*dq2*cos( q1 )*cos( q2 )*sin( q3 ) - L2*dq2*cos( q1 )*cos( q3 )*sin( q2 ) - L2*dq3*cos( q1 )*cos( q2 )*sin( q3 ) - L2*dq3*cos( q1 )*cos( q3 )*sin( q2 ) - L2*dq1*cos( q2 )*cos( q3 )*sin( q1 );

dJ= [dJ11 dJ12 dJ13;
     0    dJ22 dJ23;
     dJ31 dJ32 dJ33];
 
 invJ = pinv(J);
